simulink model "AFEsimpleModifs"  (R2013a)
settings: Solver=FixedStepDiscrete  SolverMode=SingleTasking  StartTime=0.0  StopTime=20  FixedStep=Tpas  RelTol=1e-3
values from neighbouring files (symbols this model uses):
  Freq = 50    [AFE_2L_RC_param_DT1.m]    (also in AFE_FV_Params.m; AFE_PontHPV2.m; AFEsimplepara.m; AFEsimpleparaDT1.m)
  hys = 100    [AFE_2L_RC_param_DT1.m]    (also in AFE_FV_Params.m = 150; AFE_PontHPV2.m = 150; AFEsimplepara.m = 0.1; AFEsimpleparaDT1.m)
  Lac = 8.1487e-04    (= 0.00081487)    [AFE_2L_RC_param_DT1.m]    (also in AFE_FV_Params.m; AFE_PontHPV2.m; AFEsimplepara.m; AFEsimpleparaDT1.m)
  Phase = -45    [AFEsimplepara.m]
  Rch = 9.26    [AFE_2L_RC_param_DT1.m]    (also in AFE_FV_Params.m; AFE_PontHPV2.m; AFEsimplepara.m; AFEsimpleparaDT1.m)
  Tpas = 5e-5    (= 5e-05)    [AFE_2L_RC_param_DT1.m]    (also in AFE_FV_Params.m; AFE_PontHPV2.m = 3e-06; AFEsimplepara.m; AFEsimpleparaDT1.m)
  Vac = 2000    [AFE_2L_RC_param_DT1.m]    (also in AFE_FV_Params.m; AFE_PontHPV2.m; AFEsimplepara.m; AFEsimpleparaDT1.m)
  Vdc = 5000    [AFE_2L_RC_param_DT1.m]    (also in AFE_FV_Params.m; AFE_PontHPV2.m; AFEsimplepara.m; AFEsimpleparaDT1.m)
undefined symbols (not defined in the file or in its folder): Rac
libraries: powerlib x19, powerlib_extras x3, powerlib_meascontrol x1
settings Model: Creator=LiberT  LastModifiedBy=Daniel
settings DataIOCC: SignalLoggingSaveFormat=ModelDataLogs
settings OptimizationCC: ExpressionDepthLimit=2147483647
settings DebuggingCC: MultiTaskDSMMsg=warning  MultiTaskCondExecSysMsg=none  FcnCallInpInsideContextMsg=EnableAllAsWarning  StrictBusMsg=None
settings RTWCC: IncludeERTFirstTime=on

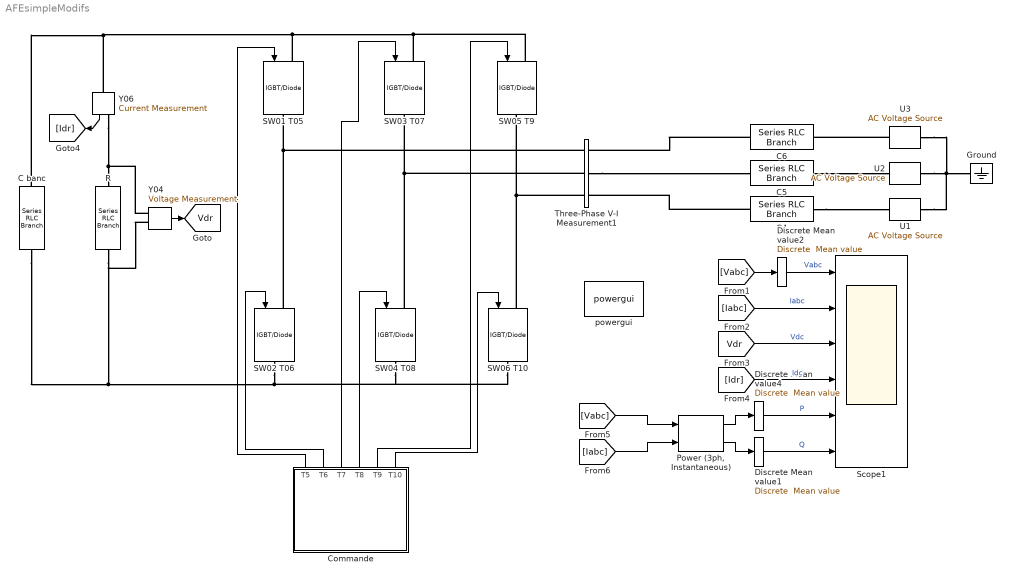
== system AFEsimpleModifs ==
  C banc : powerlib/Elements/Series RLC Branch  LConnTagsString=__new0  RConnTagsString=__new0  BranchType=C  Resistance=Rac  Inductance=Lac  SetiL0=off  InitialCurrent=0  Capacitance=300e-3  Setx0=off  InitialVoltage=5000  Measurements=None
  C4 : powerlib/Elements/Series RLC Branch  LConnTagsString=__new0  RConnTagsString=__new0  BranchType=L  Resistance=Rac  Inductance=Lac  SetiL0=off  InitialCurrent=0  Capacitance=300e-3  Setx0=off  InitialVoltage=0  Measurements=None
  C5 : powerlib/Elements/Series RLC Branch  LConnTagsString=__new0  RConnTagsString=__new0  BranchType=L  Resistance=Rac  Inductance=Lac  SetiL0=off  InitialCurrent=0  Capacitance=300e-3  Setx0=off  InitialVoltage=0  Measurements=None
  C6 : powerlib/Elements/Series RLC Branch  LConnTagsString=__new0  RConnTagsString=__new0  BranchType=L  Resistance=Rac  Inductance=Lac  SetiL0=off  InitialCurrent=0  Capacitance=300e-3  Setx0=off  InitialVoltage=0  Measurements=None
  Commande : Subsystem
  Discrete Mean value1 : powerlib_extras/Discrete Measurements/Discrete  Mean value  Freq=Freq  Vinit=0  Ts=Tpas
  Discrete Mean value2 : powerlib_extras/Discrete Measurements/Discrete  Mean value  Freq=250  Vinit=0  Ts=Tpas
  Discrete Mean value4 : powerlib_extras/Discrete Measurements/Discrete  Mean value  Freq=Freq  Vinit=0  Ts=Tpas
  Ground : powerlib/Elements/Ground  LConnTagsString=a
  "Power (3ph, Instantaneous)" : powerlib_meascontrol/Measurements/Power (3ph, Instantaneous)
  R : powerlib/Elements/Series RLC Branch  LConnTagsString=__new0  RConnTagsString=__new0  BranchType=R  Resistance=Rch  Inductance=Lac  SetiL0=off  InitialCurrent=0  Capacitance=300e-3  Setx0=off  InitialVoltage=0  Measurements=None
  SW01 T05 : powerlib/Power Electronics/IGBT//Diode  Ron=1e-3  Rs=1e5  Cs=Tpas  Measurements=off
  SW02 T06 : powerlib/Power Electronics/IGBT//Diode  Ron=1e-3  Rs=1e5  Cs=Tpas  Measurements=off
  SW03 T07 : powerlib/Power Electronics/IGBT//Diode  Ron=1e-3  Rs=1e5  Cs=Tpas  Measurements=off
  SW04 T08 : powerlib/Power Electronics/IGBT//Diode  Ron=1e-3  Rs=1e5  Cs=Tpas  Measurements=off
  SW05 T9 : powerlib/Power Electronics/IGBT//Diode  Ron=1e-3  Rs=1e5  Cs=Tpas  Measurements=off
  SW06 T10 : powerlib/Power Electronics/IGBT//Diode  Ron=1e-3  Rs=1e5  Cs=Tpas  Measurements=off
  Scope1 : Scope  NumInputPorts=6
      settings: TickLabels=on  TimeRange=0.2  YMin=-3000~-5000~4057.5~438.25~-1.8445e+06~1.431e+07  YMax=3000~5000~4075~440~-1.8405e+06~1.441e+07
  Three-Phase V-I Measurement1 : powerlib/Measurements/Three-Phase V-I Measurement  VoltageMeasurement=phase-to-ground  SetLabelV=on  LabelV=Vabc  Vpu=off  VpuLL=off  CurrentMeasurement=yes  SetLabelI=on  LabelI=Iabc  Ipu=off  Pbase=100e6  Vbase=500e3  OutputType=Complex  PhasorSimulation=off  PSBequivalent=0
  U1 : powerlib/Electrical Sources/AC Voltage Source  Amplitude=Vac*sqrt(2/3)  Phase=0  Frequency=Freq  SampleTime=0  Measurements=None
  U2 : powerlib/Electrical Sources/AC Voltage Source  Amplitude=Vac*sqrt(2/3)  Phase=120  Frequency=Freq  SampleTime=0  Measurements=None
  U3 : powerlib/Electrical Sources/AC Voltage Source  Amplitude=Vac*sqrt(2/3)  Phase=240  Frequency=Freq  SampleTime=0  Measurements=None
  Y04 : powerlib/Measurements/Voltage Measurement  PhasorSimulation=off  OutputType=Complex  PSBequivalent=0
  Y06 : powerlib/Measurements/Current Measurement  PhasorSimulation=off  OutputType=Complex  PSBequivalent=0
  powergui : powerlib/powergui  Priority=1  SimulationMode=Discrete  SolverType=Tustin  SampleTime=Tpas  frequency=60  SPID=off  DisableSnubberDevices=off  DisableRonSwitches=off  DisableVfSwitches=off  SwTol=0  Interpol=off  DisplayEquations=off  frequencyindice=50  Pbase=100e6  ErrMax=1e-4  Iterations=50  UnitsV=kV  UnitsW=MW  FunctionMessages=off  echomessages=off  HookPort=off  EnableUseOfTLC=off  x0status=blocks  RestoreLinks=warning  ResistiveCurrentMeasurement=off  Frange=[0:2:500]  Ylog=off  Xlog=on  ShowGrid=off  save=off  variable=ZData  structure=ScopeData1  ZoomFFT=off  StartTime=18  cycles=100  DisplayStyle=1  fundamental=50  FreqAxis=off  MaxFrequency=2000  frequencyindicesteady=1  RmsSteady=1  display=off  Ts=0  methode=off
  tag scope: Vdr=global
  wires:
  Y04/1 -> [Vdr]
  [Vabc] -> Discrete Mean value2/1
  [Iabc] -> Scope1/2  "Iabc"
  [Vdr] -> Scope1/3  "Vdc"
  [Idr] -> Scope1/4  "Idc"
  "Power (3ph, Instantaneous)"/1 -> Discrete Mean value4/1
  "Power (3ph, Instantaneous)"/2 -> Discrete Mean value1/1
  Discrete Mean value4/1 -> Scope1/5  "P"
  Discrete Mean value1/1 -> Scope1/6  "Q"
  [Vabc] -> "Power (3ph, Instantaneous)"/1
  [Iabc] -> "Power (3ph, Instantaneous)"/2
  Y06/1 -> [Idr]
  Commande/1(T5) -> SW01 T05/1
  Commande/2(T6) -> SW02 T06/1
  Commande/4(T8) -> SW04 T08/1
  Commande/3(T7) -> SW03 T07/1
  Commande/6(T10) -> SW06 T10/1
  Commande/5(T9) -> SW05 T9/1
  Discrete Mean value2/1 -> Scope1/1  "Vabc"
  connections:
  SW02 T06/RConn1 -- C banc/RConn1 -- Y04/LConn2 -- R/RConn1 -- SW06 T10/RConn1 -- SW04 T08/RConn1
  Y06/LConn1 -- C banc/LConn1 -- SW01 T05/LConn1 -- SW05 T9/LConn1 -- SW03 T07/LConn1
  Three-Phase V-I Measurement1/RConn2 -- C5/LConn1
  Y06/RConn1 -- Y04/LConn1 -- R/LConn1
  SW02 T06/LConn1 -- Three-Phase V-I Measurement1/LConn1 -- SW01 T05/RConn1
  SW06 T10/LConn1 -- Three-Phase V-I Measurement1/LConn3 -- SW05 T9/RConn1
  SW04 T08/LConn1 -- Three-Phase V-I Measurement1/LConn2 -- SW03 T07/RConn1
  C6/LConn1 -- Three-Phase V-I Measurement1/RConn1
  C4/LConn1 -- Three-Phase V-I Measurement1/RConn3
  U2/LConn1 -- U1/LConn1 -- U3/LConn1 -- Ground/LConn1
  C5/RConn1 -- U2/RConn1
  C4/RConn1 -- U1/RConn1
  U3/RConn1 -- C6/RConn1

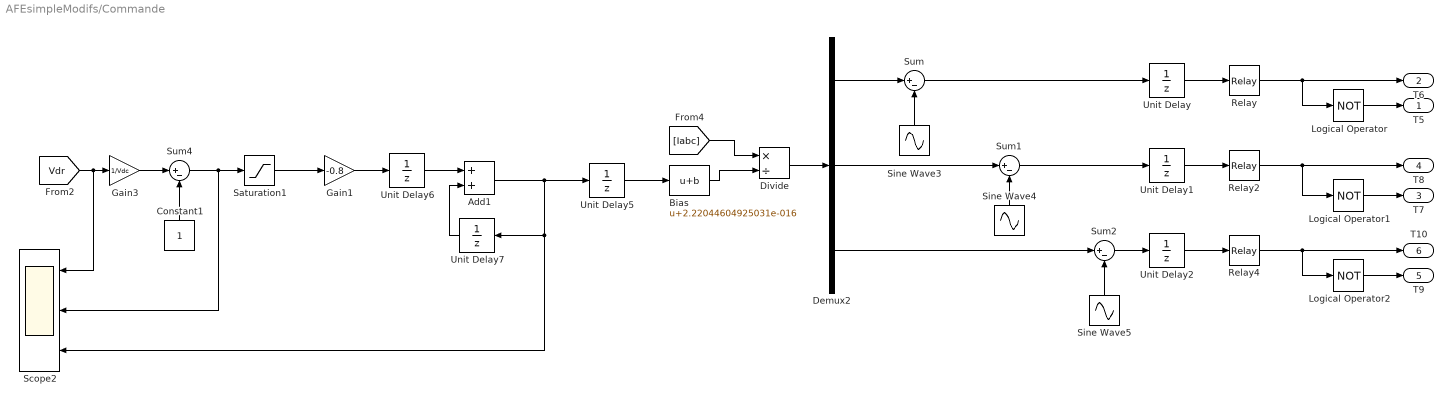
== system AFEsimpleModifs/Commande ==
  Add1 : Sum  SampleTime=Tpas
  Bias : Bias  Bias=2.22044604925031e-016
  Constant1 : Constant  SampleTime=Tpas
  Demux2 : Demux  Outputs=3
  Divide : Product  Inputs=*/  SampleTime=Tpas
  Gain1 : Gain  Gain=-0.8  SampleTime=Tpas
  Gain3 : Gain  Gain=1/Vdc  SampleTime=Tpas
  Logical Operator : Logic  Operator=NOT  AllPortsSameDT=off
  Logical Operator1 : Logic  Operator=NOT  AllPortsSameDT=off
  Logical Operator2 : Logic  Operator=NOT  AllPortsSameDT=off
  Relay : Relay  OnSwitchValue=hys  OffSwitchValue=-hys
  Relay2 : Relay  OnSwitchValue=hys  OffSwitchValue=-hys
  Relay4 : Relay  OnSwitchValue=hys  OffSwitchValue=-hys
  Saturation1 : Saturate  UpperLimit=1  LowerLimit=-1  SampleTime=Tpas
  Scope2 : Scope  NumInputPorts=3
      settings: TickLabels=on  TimeRange=0.2  YMin=-1~4966~-0.0068  YMax=1~4972~-0.0056  SaveName=ScopeData2
  Sine Wave3 : Sin  Frequency=Freq*2*pi  Phase=(Phase+240)*2*pi/360  SampleTime=0
  Sine Wave4 : Sin  Frequency=Freq*2*pi  Phase=(Phase+120)*2*pi/360  SampleTime=0
  Sine Wave5 : Sin  Frequency=Freq*2*pi  Phase=(Phase)*2*pi/360  SampleTime=0
  Sum : Sum  Inputs=|+-
  Sum1 : Sum  Inputs=|+-
  Sum2 : Sum  Inputs=|+-
  Sum4 : Sum  Inputs=|+-  SampleTime=Tpas
  Unit Delay{,1..2,5} (4 alike) : UnitDelay  SampleTime=-1
  Unit Delay6 : UnitDelay  SampleTime=Tpas
  Unit Delay7 : UnitDelay  SampleTime=Tpas
  T5 : Outport
  T6 : Outport  Port=2
  T7 : Outport  Port=3
  T8 : Outport  Port=4
  T9 : Outport  Port=5
  T10 : Outport  Port=6
  wires:
  Demux2/1 -> Sum/1
  Demux2/2 -> Sum1/1
  Demux2/3 -> Sum2/1
  Sum/1 -> Unit Delay/1
  Sum1/1 -> Unit Delay1/1
  Sum2/1 -> Unit Delay2/1
  Unit Delay/1 -> Relay/1
  Unit Delay1/1 -> Relay2/1
  Unit Delay2/1 -> Relay4/1
  Logical Operator/1 -> T5/1
  Logical Operator1/1 -> T7/1
  Logical Operator2/1 -> T9/1
  Relay/1 -> T6/1, Logical Operator/1
  Relay2/1 -> T8/1, Logical Operator1/1
  Relay4/1 -> T10/1, Logical Operator2/1
  [Iabc] -> Divide/1
  [Vdr] -> Scope2/1, Gain3/1
  Gain3/1 -> Sum4/1
  Constant1/1 -> Sum4/2
  Sum4/1 -> Scope2/2, Saturation1/1
  Saturation1/1 -> Gain1/1
  Gain1/1 -> Unit Delay6/1
  Unit Delay7/1 -> Add1/2
  Unit Delay6/1 -> Add1/1
  Add1/1 -> Scope2/3, Unit Delay7/1, Unit Delay5/1
  Sine Wave3/1 -> Sum/2
  Sine Wave4/1 -> Sum1/2
  Sine Wave5/1 -> Sum2/2
  Divide/1 -> Demux2/1
  Unit Delay5/1 -> Bias/1
  Bias/1 -> Divide/2
